simulink model "untitled"  (R2020b)
settings: Solver=FixedStepDiscrete  StartTime=0.0  StopTime=10.0  FixedStep=0.0001  RelTol=1e-3  EnableMultiTasking=on
libraries: simulink x1
settings Model: Creator=LYX  LastModifiedBy=LYX

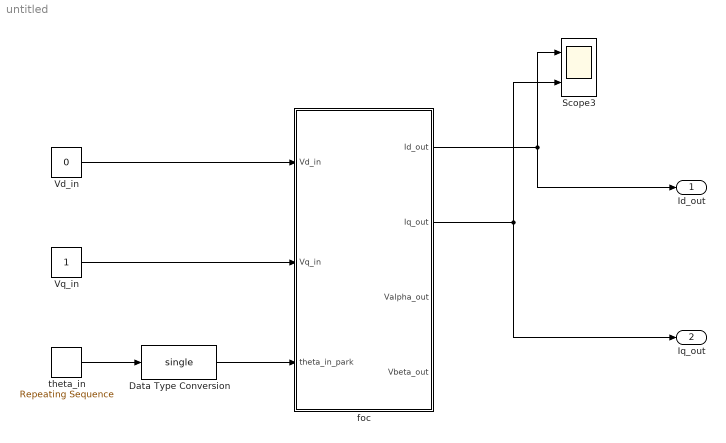
== system untitled ==
  Data Type Conversion : DataTypeConversion  OutDataTypeStr=single
  Scope3 : Scope  NumInputPorts=2
  Vd_in : Constant  Value=0  OutDataTypeStr=single
  Vq_in : Constant  OutDataTypeStr=single
  foc : Subsystem
  theta_in : simulink/Sources/Repeating Sequence  rep_seq_t=[0 0.1]  rep_seq_y=[0 2*pi]
  Id_out : Outport
  Iq_out : Outport  Port=2
  wires:
  foc/2(Iq_out) -> Iq_out/1, Scope3/2
  foc/1(Id_out) -> Id_out/1, Scope3/1
  Vd_in/1 -> foc/1(Vd_in)
  Vq_in/1 -> foc/2(Vq_in)
  theta_in/1 -> Data Type Conversion/1
  Data Type Conversion/1 -> foc/3(theta_in_park)

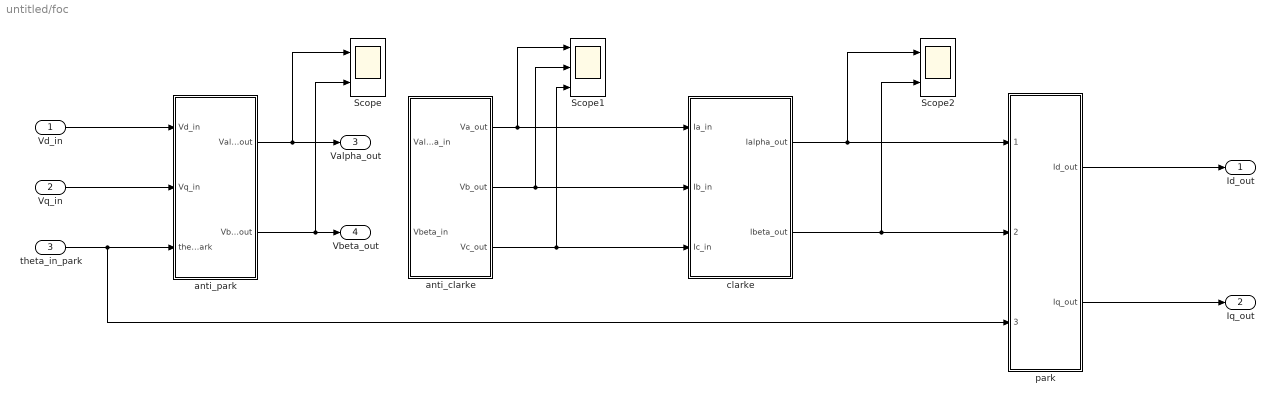
== system untitled/foc ==
  Vd_in : Inport
  Vq_in : Inport  Port=2
  theta_in_park : Inport  Port=3
  Scope : Scope  NumInputPorts=2
  Scope1 : Scope  NumInputPorts=3
  Scope2 : Scope  NumInputPorts=2
  anti_clarke : Subsystem
  anti_park : Subsystem
  clarke : Subsystem
  park : Subsystem
  Id_out : Outport
  Iq_out : Outport  Port=2
  Valpha_out : Outport  Port=3
  Vbeta_out : Outport  Port=4
  wires:
  Vd_in/1 -> anti_park/1(Vd_in)
  anti_clarke/1(Va_out) -> clarke/1(Ia_in), Scope1/1
  anti_park/1(Valpha_out) -> Valpha_out/1, Scope/1
  theta_in_park/1 -> park/3(theta_in_park), anti_park/3(theta_in_antipark)
  anti_clarke/2(Vb_out) -> clarke/2(Ib_in), Scope1/2
  park/1(Id_out) -> Id_out/1
  anti_park/2(Vbeta_out) -> Vbeta_out/1, Scope/2
  anti_clarke/3(Vc_out) -> clarke/3(Ic_in), Scope1/3
  clarke/2(Ibeta_out) -> Scope2/2, park/2(Ibeta_in)
  clarke/1(Ialpha_out) -> Scope2/1, park/1(Ialpha_in)
  Vq_in/1 -> anti_park/2(Vq_in)
  park/2(Iq_out) -> Iq_out/1

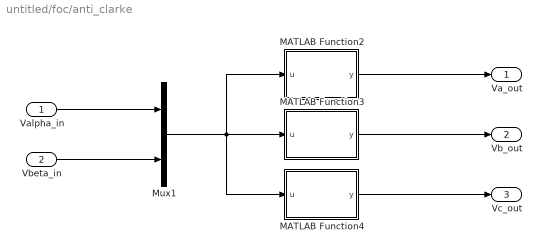
== system untitled/foc/anti_clarke ==
  Valpha_in : Inport
  Vbeta_in : Inport  Port=2
  MATLAB Function2 : MATLAB Function  TreatAsAtomicUnit=on
  MATLAB Function3 : MATLAB Function  TreatAsAtomicUnit=on
  MATLAB Function4 : MATLAB Function  TreatAsAtomicUnit=on
  Mux1 : Mux  Inputs=2
  Va_out : Outport
  Vb_out : Outport  Port=2
  Vc_out : Outport  Port=3
  wires:
  MATLAB Function2/1(y) -> Va_out/1
  Valpha_in/1 -> Mux1/1
  Vbeta_in/1 -> Mux1/2
  Mux1/1 -> MATLAB Function4/1(u), MATLAB Function3/1(u), MATLAB Function2/1(u)
  MATLAB Function3/1(y) -> Vb_out/1
  MATLAB Function4/1(y) -> Vc_out/1

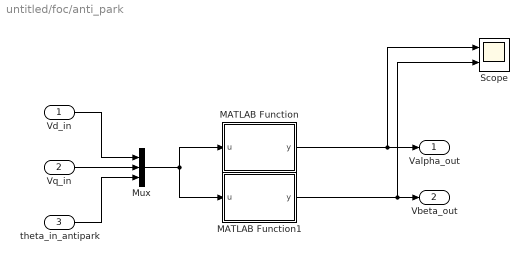
== system untitled/foc/anti_park ==
  Vd_in : Inport
  Vq_in : Inport  Port=2
  theta_in_antipark : Inport  Port=3
  MATLAB Function : MATLAB Function  TreatAsAtomicUnit=on
  MATLAB Function1 : MATLAB Function  TreatAsAtomicUnit=on
  Mux : Mux  Inputs=3
  Scope : Scope  NumInputPorts=2
  Valpha_out : Outport
  Vbeta_out : Outport  Port=2
  wires:
  Mux/1 -> MATLAB Function1/1(u), MATLAB Function/1(u)
  theta_in_antipark/1 -> Mux/3
  Vq_in/1 -> Mux/2
  Vd_in/1 -> Mux/1
  MATLAB Function/1(y) -> Scope/1, Valpha_out/1
  MATLAB Function1/1(y) -> Scope/2, Vbeta_out/1

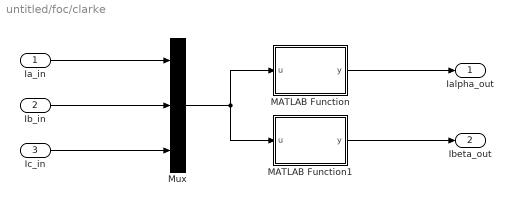
== system untitled/foc/clarke ==
  Ia_in : Inport
  Ib_in : Inport  Port=2
  Ic_in : Inport  Port=3
  MATLAB Function : MATLAB Function  TreatAsAtomicUnit=on
  MATLAB Function1 : MATLAB Function  TreatAsAtomicUnit=on
  Mux : Mux  Inputs=3
  Ialpha_out : Outport
  Ibeta_out : Outport  Port=2
  wires:
  Ib_in/1 -> Mux/2
  Mux/1 -> MATLAB Function1/1(u), MATLAB Function/1(u)
  Ia_in/1 -> Mux/1
  MATLAB Function1/1(y) -> Ibeta_out/1
  MATLAB Function/1(y) -> Ialpha_out/1
  Ic_in/1 -> Mux/3

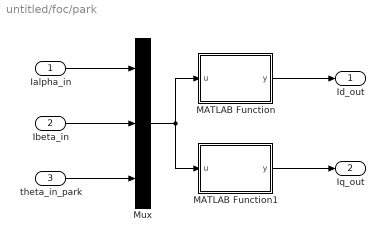
== system untitled/foc/park ==
  Ialpha_in : Inport
  Ibeta_in : Inport  Port=2
  theta_in_park : Inport  Port=3
  MATLAB Function : MATLAB Function  TreatAsAtomicUnit=on
  MATLAB Function1 : MATLAB Function  TreatAsAtomicUnit=on
  Mux : Mux  Inputs=3
  Id_out : Outport
  Iq_out : Outport  Port=2
  wires:
  Ialpha_in/1 -> Mux/1
  Mux/1 -> MATLAB Function1/1(u), MATLAB Function/1(u)
  MATLAB Function1/1(y) -> Iq_out/1
  Ibeta_in/1 -> Mux/2
  theta_in_park/1 -> Mux/3
  MATLAB Function/1(y) -> Id_out/1

== matlab function untitled/foc/anti_park/MATLAB Function ==
  data: u input; y output
function y = fcn(u)

y = u(1)*cos(u(3))-u(2)*sin(u(3));

== matlab function untitled/foc/anti_clarke/MATLAB Function2 ==
  data: u input; y output
function y = fcn(u)

y = u(1);

== matlab function untitled/foc/anti_clarke/MATLAB Function3 ==
  data: u input; y output
function y = fcn(u)

y = (-u(1)+sqrt(3)*u(2))/2;

== matlab function untitled/foc/anti_clarke/MATLAB Function4 ==
  data: u input; y output
function y = fcn(u)

y = (-u(1)-sqrt(3)*u(2))/2;

== matlab function untitled/foc/clarke/MATLAB Function ==
  data: u input; y output
function y = fcn(u)

y = u(1);

== matlab function untitled/foc/clarke/MATLAB Function1 ==
  data: u input; y output
function y = fcn(u)

y = (u(1)+2*u(2))/sqrt(3);

== matlab function untitled/foc/park/MATLAB Function ==
  data: u input; y output
function y = fcn(u)

y = u(1)*cos(u(3))+u(2)*sin(u(3));

== matlab function untitled/foc/park/MATLAB Function1 ==
  data: u input; y output
function y = fcn(u)

y = -u(1)*sin(u(3))+u(2)*cos(u(3))

== matlab function untitled/foc/anti_park/MATLAB Function1 ==
  data: u input; y output
function y = fcn(u)

y = u(1)*sin(u(3))+u(2)*cos(u(3));
